simulink model "inverted_pendulum_on_cart"  (R2019a)
settings: Solver=VariableStepAuto  StartTime=0.0  StopTime=10.0  RelTol=1e-3
values from neighbouring files (symbols this model uses):
  b = 0.1    [Inverted_pendulum_on_cart.mat]
  g = 9.8    [Inverted_pendulum_on_cart.mat]
  I = 0.006    [Inverted_pendulum_on_cart.mat]
  l = 0.3    [Inverted_pendulum_on_cart.mat]
  M = 0.5    [Inverted_pendulum_on_cart.mat]
  m = 0.2    [Inverted_pendulum_on_cart.mat]
libraries: simulink x2
settings Model: Creator=Ranish  LastModifiedBy=Ranish

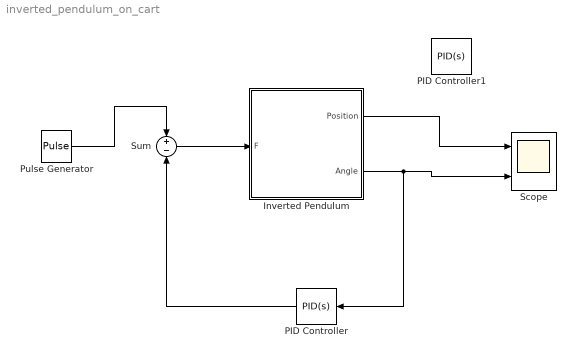
== system inverted_pendulum_on_cart ==
  "Inverted Pendulum " : Subsystem
  PID Controller : simulink/Continuous/PID Controller  Controller=PID  Form=Parallel  TimeDomain=Continuous-time  SampleTime=-1  IntegratorMethod=Forward Euler  FilterMethod=Forward Euler  ControllerParametersSource=internal  P=100  I=1  D=21  UseFilter=on  N=100  TunerSelectOption=Transfer Function Based (PID Tuner App)  InitialConditionSource=internal  InitialConditionForIntegrator=0  InitialConditionForFilter=0  DifferentiatorICPrevScaledInput=0  ExternalReset=none  TrackingMode=off  Kt=1  LimitOutput=off  UpperSaturationLimit=inf  LowerSaturationLimit=-inf  LinearizeAsGain=on  AntiWindupMode=none  Kb=1  POutMin=[]  POutMax=[]  IOutMin=[]  IOutMax=[]  DOutMin=[]  DOutMax=[]  NOutMin=[]  NOutMax=[]  SumOutMin=[]  SumOutMax=[]  SaturationOutMin=[]  SaturationOutMax=[]  PParamMin=[]  PParamMax=[]  IParamMin=[]  IParamMax=[]  DParamMin=[]  DParamMax=[]  NParamMin=[]  NParamMax=[]  KbParamMin=[]  KbParamMax=[]  KtParamMin=[]  KtParamMax=[]  KbOutMin=[]  KbOutMax=[]  KtOutMin=[]  KtOutMax=[]  IntegratorOutMin=[]  IntegratorOutMax=[]  FilterOutMin=[]  FilterOutMax=[]  SumI1OutMin=[]  SumI1OutMax=[]  SumI2OutMin=[]  SumI2OutMax=[]  SumI3OutMin=[]  SumI3OutMax=[]  SumI4OutMin=[]  SumI4OutMax=[]  SumDOutMin=[]  SumDOutMax=[]  DifferentiatorOutMin=[]  DifferentiatorOutMax=[]  FilterDiffOutCoefMin=[]  FilterDiffOutCoefMax=[]  ReciprocalOutMin=[]  ReciprocalOutMax=[]  SumDenOutMin=[]  SumDenOutMax=[]  SumNumOutMin=[]  SumNumOutMax=[]  DivideOutMin=[]  DivideOutMax=[]  IntegratorContinuousStateAttributes=''  IntegratorStateMustResolveToSignalObject=off  IntegratorRTWStateStorageClass=Auto  FilterContinuousStateAttributes=''  FilterStateMustResolveToSignalObject=off  FilterRTWStateStorageClass=Auto  ParallelPVariant=InternalParameters  IdealPVariant=Disabled  IVariant=InternalParameters  DVariant=InternalParameters  IntegratorVariant=Continuous  SatVariant=Disabled  AWVariant=Passthrough  PCopyVariant=Disabled  TRVariant=Disabled  FdbkBlocksVariant=Forward  IdealPFdbkVariant=Disabled  SatFdbkVariant=Disabled  DerivativeFilterVariant=ContFilter  NVariant=InternalParameters  NCopyVariant=Disabled  FilterICVariant=InternalICsFilter  IntegratorICVariant=InternalICs  ExternalResetVariant=Disabled  TRSumVariant=Passthrough  SumFdbkVariant=Disabled  SumVariant=Sum_PID
  PID Controller1 : simulink/Continuous/PID Controller  Controller=PID  Form=Parallel  TimeDomain=Continuous-time  SampleTime=-1  IntegratorMethod=Forward Euler  FilterMethod=Forward Euler  ControllerParametersSource=internal  P=1  I=1  D=0  UseFilter=on  N=100  TunerSelectOption=Transfer Function Based (PID Tuner App)  InitialConditionSource=internal  InitialConditionForIntegrator=0  InitialConditionForFilter=0  DifferentiatorICPrevScaledInput=0  ExternalReset=none  TrackingMode=off  Kt=1  LimitOutput=off  UpperSaturationLimit=inf  LowerSaturationLimit=-inf  LinearizeAsGain=on  AntiWindupMode=none  Kb=1  POutMin=[]  POutMax=[]  IOutMin=[]  IOutMax=[]  DOutMin=[]  DOutMax=[]  NOutMin=[]  NOutMax=[]  SumOutMin=[]  SumOutMax=[]  SaturationOutMin=[]  SaturationOutMax=[]  PParamMin=[]  PParamMax=[]  IParamMin=[]  IParamMax=[]  DParamMin=[]  DParamMax=[]  NParamMin=[]  NParamMax=[]  KbParamMin=[]  KbParamMax=[]  KtParamMin=[]  KtParamMax=[]  KbOutMin=[]  KbOutMax=[]  KtOutMin=[]  KtOutMax=[]  IntegratorOutMin=[]  IntegratorOutMax=[]  FilterOutMin=[]  FilterOutMax=[]  SumI1OutMin=[]  SumI1OutMax=[]  SumI2OutMin=[]  SumI2OutMax=[]  SumI3OutMin=[]  SumI3OutMax=[]  SumI4OutMin=[]  SumI4OutMax=[]  SumDOutMin=[]  SumDOutMax=[]  DifferentiatorOutMin=[]  DifferentiatorOutMax=[]  FilterDiffOutCoefMin=[]  FilterDiffOutCoefMax=[]  ReciprocalOutMin=[]  ReciprocalOutMax=[]  SumDenOutMin=[]  SumDenOutMax=[]  SumNumOutMin=[]  SumNumOutMax=[]  DivideOutMin=[]  DivideOutMax=[]  IntegratorContinuousStateAttributes=''  IntegratorStateMustResolveToSignalObject=off  IntegratorRTWStateStorageClass=Auto  FilterContinuousStateAttributes=''  FilterStateMustResolveToSignalObject=off  FilterRTWStateStorageClass=Auto  ParallelPVariant=InternalParameters  IdealPVariant=Disabled  IVariant=InternalParameters  DVariant=InternalParameters  IntegratorVariant=Continuous  SatVariant=Disabled  AWVariant=Passthrough  PCopyVariant=Disabled  TRVariant=Disabled  FdbkBlocksVariant=Forward  IdealPFdbkVariant=Disabled  SatFdbkVariant=Disabled  DerivativeFilterVariant=ContFilter  NVariant=InternalParameters  NCopyVariant=Disabled  FilterICVariant=InternalICsFilter  IntegratorICVariant=InternalICs  ExternalResetVariant=Disabled  TRSumVariant=Passthrough  SumFdbkVariant=Disabled  SumVariant=Sum_PID
  Pulse Generator : DiscretePulseGenerator  PulseType=Time based  Amplitude=1000  Period=10  PulseWidth=0.1
  Scope : Scope  NumInputPorts=2
  Sum : Sum  Inputs=+-
  wires:
  "Inverted Pendulum "/1(Position) -> Scope/1
  "Inverted Pendulum "/2(Angle) -> PID Controller/1, Scope/2
  Pulse Generator/1 -> Sum/1
  Sum/1 -> "Inverted Pendulum "/1(F)
  PID Controller/1 -> Sum/2

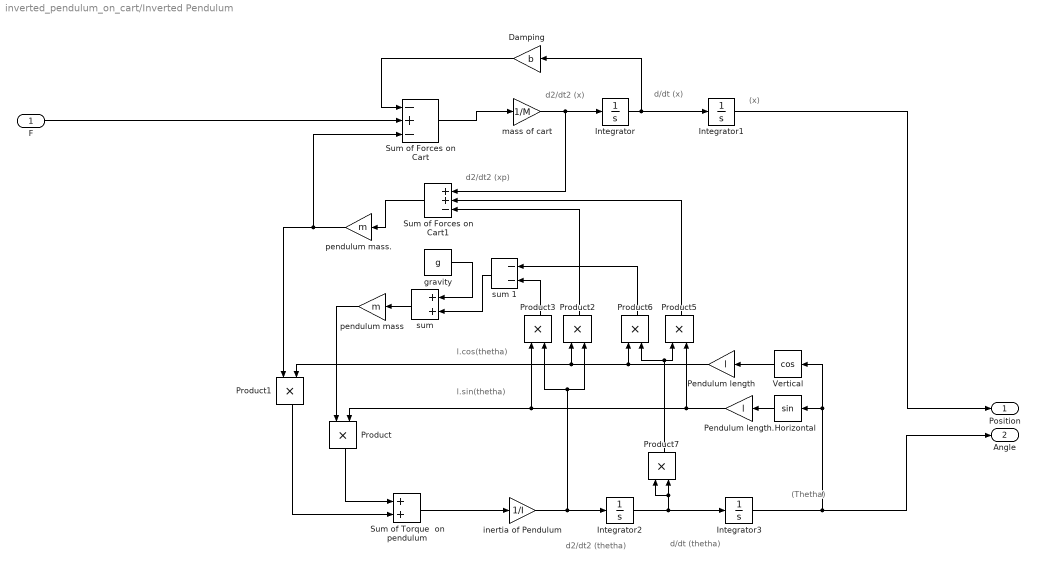
== system inverted_pendulum_on_cart/Inverted Pendulum  ==
  note: l.cos(thetha)
  note: (Thetha)
  note: (x)
  note: d/dt (thetha)
  note: d2/dt2 (thetha)
  note: d/dt (x)
  note: d2/dt2 (x)
  note: d2/dt2 (xp)
  note: l.sin(thetha)
  F : Inport
  Damping : Gain  Gain=b
  Horizontal : Trigonometry
  Integrator{,1..3} (4 alike) : Integrator
  Pendulum length : Gain  Gain=l
  Pendulum length. : Gain  Gain=l
  Product{,1..3,5..7} (7 alike) : Product
  Sum of Forces on Cart : Sum  Inputs=-+-
  Sum of Forces on Cart1 : Sum  Inputs=++-
  Sum of Torque  on pendulum : Sum
  Vertical : Trigonometry  Operator=cos
  gravity : Constant  Value=g
  "inertia of Pendulum " : Gain  Gain=1/I
  mass of cart : Gain  Gain=1/M
  "pendulum mass " : Gain  Gain=m
  "pendulum mass. " : Gain  Gain=m
  "sum " : Sum
  sum 1 : Sum  Inputs=--
  Position : Outport
  Angle : Outport  Port=2
  wires:
  "inertia of Pendulum "/1 -> Integrator2/1, Product3/2, Product2/2
  Product/1 -> Sum of Torque  on pendulum/1
  Integrator3/1 -> Angle/1, Horizontal/1, Vertical/1
  Pendulum length/1 -> Product2/1, Product1/2, Product6/1
  Horizontal/1 -> Pendulum length./1
  Sum of Forces on Cart1/1 -> "pendulum mass. "/1
  Integrator/1 -> Damping/1, Integrator1/1
  Pendulum length./1 -> Product3/1, Product/2, Product5/2
  "pendulum mass. "/1 -> Sum of Forces on Cart/3, Product1/1
  Product6/1 -> sum 1/1
  Damping/1 -> Sum of Forces on Cart/1
  mass of cart/1 -> Sum of Forces on Cart1/1, Integrator/1
  F/1 -> Sum of Forces on Cart/2
  Product1/1 -> Sum of Torque  on pendulum/2
  Sum of Torque  on pendulum/1 -> "inertia of Pendulum "/1
  "sum "/1 -> "pendulum mass "/1
  Product5/1 -> Sum of Forces on Cart1/2
  Integrator2/1 -> Integrator3/1, Product7/1, Product7/2
  Product7/1 -> Product5/1, Product6/2
  Product2/1 -> Sum of Forces on Cart1/3
  "pendulum mass "/1 -> Product/1
  Vertical/1 -> Pendulum length/1
  Sum of Forces on Cart/1 -> mass of cart/1
  Integrator1/1 -> Position/1
  sum 1/1 -> "sum "/2
  gravity/1 -> "sum "/1
  Product3/1 -> sum 1/2
